simulink model "KUKA_AdaptiveComputedTorque"  (R2021a)
settings: Solver=FixedStepAuto  StartTime=0.0  StopTime=4  FixedStep=0.001  RelTol=1e-3
InitFcn:
  | Gamma=eye(8)*0.1;
  | K=[8100 900 6400 6400;180 60 160 160];
values from neighbouring files (symbols this model uses):
  m = {0 0 0 0 0}    [DynMatrixCalculator.m]
  N = {zeros(3,1) zeros(3,1) zeros(3,1) zeros(3,1) zeros(3,1)}    [DynMatrixCalculator.m]
undefined symbols (not defined in the file or in its folder): X, Y, Z
libraries: nesl_utility x17, sm_lib x16
(part 2 of 2)

== matlab function KUKA_AdaptiveComputedTorque/MATLAB Function1 ==
  data: Gamma input; K input; Theta_dd_ref input; Error input; Error_d input; Theta_dd input; Theta_d input; Theta input; Phi input; Tau output; Phi_hat_d output
function [Tau,Phi_hat_d] = Controller(Gamma,K,Theta_dd_ref, Error,Error_d,Theta_dd,Theta_d,Theta,Phi)

%% Input Data
d=Theta(1);
th2=Theta(2);
th3=Theta(3);
th4=Theta(4);

d_dt=Theta_d(1);
th2_dt=Theta_d(2);
th3_dt=Theta_d(3);
th4_dt=Theta_d(4);

d_ddt=Theta_dd(1);
th2_ddt=Theta_dd(2);
th3_ddt=Theta_dd(3);
th4_ddt=Theta_dd(4);


m1=Phi(1);m2=Phi(2);m3=Phi(3);m4=Phi(4);
I1=Phi(5);I2=Phi(6);I3=Phi(7);I4=Phi(8);
%% Params
g=9.80665;
% Kp = diag([100 100 100 100]);
% % ki = diag([2 4 4 4]);
% Kv = diag([20 20 20 20]);

Kp=diag(K(1,:));
% Ki=diag(K(2,:));
Kv=diag(K(2,:));

%% MVG
M =[                                                                                                                                                                                                                                                                                                                                                                                                        m1 + m2 + m3 + m4, (m2*cos(th2))/200 - (m2*sin(th2))/1000 + (m3*sin(th2))/1000 + (m4*sin(th2))/1000 + (11*m3*cos(th2)*cos(th3))/1000 + (59*m3*cos(th2)*sin(th3))/500 + (29*m4*cos(th2)*sin(th3))/100 - (143*m4*cos(th2)*cos(th3)*cos(th4))/1000 + (3*m4*cos(th2)*cos(th3)*sin(th4))/200 + (3*m4*cos(th2)*cos(th4)*sin(th3))/200 + (143*m4*cos(th2)*sin(th3)*sin(th4))/1000,                                                                                                                              sin(th2)*((59*m3*cos(th3))/500 + (29*m4*cos(th3))/100 - (11*m3*sin(th3))/1000 + (3*m4*cos(th3 + th4))/200 + (143*m4*sin(th3 + th4))/1000),             (20674^(1/2)*m4*sin(atan(15/143) + th3 + th4)*sin(th2))/1000
(m2*cos(th2))/200 - (m2*sin(th2))/1000 + (m3*sin(th2))/1000 + (m4*sin(th2))/1000 + (11*m3*cos(th2)*cos(th3))/1000 + (59*m3*cos(th2)*sin(th3))/500 + (29*m4*cos(th2)*sin(th3))/100 - (143*m4*cos(th2)*cos(th3)*cos(th4))/1000 + (3*m4*cos(th2)*cos(th3)*sin(th4))/200 + (3*m4*cos(th2)*cos(th4)*sin(th3))/200 + (143*m4*cos(th2)*sin(th3)*sin(th4))/1000,                 I2 + I3 + I4 + (13*m2)/500000 + (14047*m3)/2000000 + (13097*m4)/250000 + (87*m4*cos(th4))/20000 + (158*m4*cos(2*th3 + 2*th4))/15625 + (4147*m4*sin(th4))/100000 - (429*m4*sin(2*th3 + 2*th4))/200000 - (13803*m3*cos(2*th3))/2000000 - (841*m4*cos(2*th3))/20000 + (649*m3*sin(2*th3))/500000 - (87*m4*cos(2*th3 + th4))/20000 - (4147*m4*sin(2*th3 + th4))/100000, cos(th3)*((59*m3)/500000 + (m4*cos(th4)*((29*cos(th4))/100 + 3/200))/1000 + (m4*sin(th4)*((29*sin(th4))/100 + 143/1000))/1000) - sin(th3)*((11*m3)/1000000 + (m4*sin(th4)*((29*cos(th4))/100 + 3/200))/1000 - (m4*cos(th4)*((29*sin(th4))/100 + 143/1000))/1000),                      (20674^(1/2)*m4*sin(atan(15/143) + th3 + th4))/1000000
                                                                                                                                                                                                                                                                              (sin(th2)*(118*m3*cos(th3) + 290*m4*cos(th3) - 11*m3*sin(th3) + 15*m4*cos(th3 + th4) + 143*m4*sin(th3 + th4)))/1000,                                                                                                                                                                                                                                                        (59*m3*cos(th3))/500000 + (29*m4*cos(th3))/100000 - (11*m3*sin(th3))/1000000 + (3*m4*cos(th3 + th4))/200000 + (143*m4*sin(th3 + th4))/1000000,                                                                                                                                                                                       I3 + I4 + (2809*m3)/200000 + (52387*m4)/500000 + (87*m4*cos(th4))/10000 + (4147*m4*sin(th4))/50000, I4 + (10337*m4)/500000 + (87*m4*cos(th4))/20000 + (4147*m4*sin(th4))/100000
                                                                                                                                                                                                                                                                                                                                                    (20674^(1/2)*m4*sin(atan(15/143) + th3 + th4)*sin(th2))/1000,                                                                                                                                                                                                                                                                                                                                                (3*m4*cos(th3 + th4))/200000 + (143*m4*sin(th3 + th4))/1000000,                                                                                                                                                                                                              I4 + (10337*m4)/500000 + (87*m4*cos(th4))/20000 + (4147*m4*sin(th4))/100000,                                                            I4 + (10337*m4)/500000];

G =[                                                                                                                                                            0
                                                                                                                                                            0
(143*g*m4*cos(th3 + th4))/1000 - (59*g*m3*sin(th3))/500 - (29*g*m4*sin(th3))/100 - (11*g*m3*cos(th3))/1000 - (3*g*m4*sin(th3 + th4))/200
                                                                                                  (20674^(1/2)*g*m4*cos(atan(15/143) + th3 + th4))/1000];
 

                                                                                                  
W=[d_ddt, d_ddt + (th2_ddt*cos(th2))/200 - (th2_ddt*sin(th2))/1000 - (th2_dt^2*cos(th2))/1000 - (th2_dt^2*sin(th2))/200,                     d_ddt + (th2_ddt*sin(th2))/1000 + (th2_dt^2*cos(th2))/1000 + (11*th2_ddt*cos(th2)*cos(th3))/1000 + (59*th2_ddt*cos(th2)*sin(th3))/500 + (59*th3_ddt*cos(th3)*sin(th2))/500 - (11*th3_ddt*sin(th2)*sin(th3))/1000 - (11*th2_dt^2*cos(th3)*sin(th2))/1000 - (11*th3_dt^2*cos(th3)*sin(th2))/1000 - (59*th2_dt^2*sin(th2)*sin(th3))/500 - (59*th3_dt^2*sin(th2)*sin(th3))/500 + (59*th2_dt*th3_dt*cos(th2)*cos(th3))/250 - (11*th2_dt*th3_dt*cos(th2)*sin(th3))/500, d_ddt + (th2_ddt*sin(th2))/1000 + (th2_dt^2*cos(th2))/1000 + (29*th2_ddt*cos(th2)*sin(th3))/100 + (29*th3_ddt*cos(th3)*sin(th2))/100 - (29*th2_dt^2*sin(th2)*sin(th3))/100 - (29*th3_dt^2*sin(th2)*sin(th3))/100 - (3*th3_ddt*sin(th2)*sin(th3)*sin(th4))/200 - (3*th4_ddt*sin(th2)*sin(th3)*sin(th4))/200 + (143*th2_dt^2*cos(th3)*cos(th4)*sin(th2))/1000 + (143*th3_dt^2*cos(th3)*cos(th4)*sin(th2))/1000 + (143*th4_dt^2*cos(th3)*cos(th4)*sin(th2))/1000 - (3*th2_dt^2*cos(th3)*sin(th2)*sin(th4))/200 - (3*th2_dt^2*cos(th4)*sin(th2)*sin(th3))/200 - (3*th3_dt^2*cos(th3)*sin(th2)*sin(th4))/200 - (3*th3_dt^2*cos(th4)*sin(th2)*sin(th3))/200 - (3*th4_dt^2*cos(th3)*sin(th2)*sin(th4))/200 - (3*th4_dt^2*cos(th4)*sin(th2)*sin(th3))/200 - (143*th2_dt^2*sin(th2)*sin(th3)*sin(th4))/1000 - (143*th3_dt^2*sin(th2)*sin(th3)*sin(th4))/1000 - (143*th4_dt^2*sin(th2)*sin(th3)*sin(th4))/1000 + (29*th2_dt*th3_dt*cos(th2)*cos(th3))/50 - (143*th2_ddt*cos(th2)*cos(th3)*cos(th4))/1000 + (3*th2_ddt*cos(th2)*cos(th3)*sin(th4))/200 + (3*th2_ddt*cos(th2)*cos(th4)*sin(th3))/200 + (3*th3_ddt*cos(th3)*cos(th4)*sin(th2))/200 + (3*th4_ddt*cos(th3)*cos(th4)*sin(th2))/200 + (143*th2_ddt*cos(th2)*sin(th3)*sin(th4))/1000 + (143*th3_ddt*cos(th3)*sin(th2)*sin(th4))/1000 + (143*th3_ddt*cos(th4)*sin(th2)*sin(th3))/1000 + (143*th4_ddt*cos(th3)*sin(th2)*sin(th4))/1000 + (143*th4_ddt*cos(th4)*sin(th2)*sin(th3))/1000 + (3*th2_dt*th3_dt*cos(th2)*cos(th3)*cos(th4))/100 + (3*th2_dt*th4_dt*cos(th2)*cos(th3)*cos(th4))/100 + (143*th2_dt*th3_dt*cos(th2)*cos(th3)*sin(th4))/500 + (143*th2_dt*th3_dt*cos(th2)*cos(th4)*sin(th3))/500 + (143*th2_dt*th4_dt*cos(th2)*cos(th3)*sin(th4))/500 + (143*th2_dt*th4_dt*cos(th2)*cos(th4)*sin(th3))/500 + (143*th3_dt*th4_dt*cos(th3)*cos(th4)*sin(th2))/500 - (3*th2_dt*th3_dt*cos(th2)*sin(th3)*sin(th4))/100 - (3*th2_dt*th4_dt*cos(th2)*sin(th3)*sin(th4))/100 - (3*th3_dt*th4_dt*cos(th3)*sin(th2)*sin(th4))/100 - (3*th3_dt*th4_dt*cos(th4)*sin(th2)*sin(th3))/100 - (143*th3_dt*th4_dt*sin(th2)*sin(th3)*sin(th4))/500, 0,      0,      0,               0
     0,                                        (13*th2_ddt)/500000 + (d_ddt*cos(th2))/200 - (d_ddt*sin(th2))/1000, (14047*th2_ddt)/2000000 + (11*d_ddt*cos(th2 + th3))/2000 + (59*d_ddt*sin(th2 + th3))/1000 + (59*th3_ddt*cos(th3))/500000 + (d_ddt*sin(th2))/1000 - (11*th3_ddt*sin(th3))/1000000 + (11*d_ddt*cos(th2 - th3))/2000 - (59*d_ddt*sin(th2 - th3))/1000 - (13803*th2_ddt*cos(2*th3))/2000000 - (11*th3_dt^2*cos(th3))/1000000 + (649*th2_ddt*sin(2*th3))/500000 - (59*th3_dt^2*sin(th3))/500000 + (649*th2_dt*th3_dt*cos(2*th3))/250000 + (13803*th2_dt*th3_dt*sin(2*th3))/1000000,                                                                                                                                                                                                                                                                                                                                                                                                                                                                                                                                             (13097*th2_ddt)/250000 + (3*th3_ddt*cos(th3 + th4))/200000 + (3*th4_ddt*cos(th3 + th4))/200000 + (29*d_ddt*sin(th2 + th3))/200 + (143*th3_ddt*sin(th3 + th4))/1000000 + (143*th4_ddt*sin(th3 + th4))/1000000 + (87*th2_ddt*cos(th4))/20000 + (29*th3_ddt*cos(th3))/100000 - (143*d_ddt*cos(th2 + th3 + th4))/2000 + (d_ddt*sin(th2))/1000 + (4147*th2_ddt*sin(th4))/100000 - (87*th2_ddt*cos(2*th3 + th4))/20000 + (143*th3_dt^2*cos(th3 + th4))/1000000 + (143*th4_dt^2*cos(th3 + th4))/1000000 + (3*d_ddt*sin(th2 + th3 + th4))/400 - (29*d_ddt*sin(th2 - th3))/200 - (4147*th2_ddt*sin(2*th3 + th4))/100000 - (3*th3_dt^2*sin(th3 + th4))/200000 - (3*th4_dt^2*sin(th3 + th4))/200000 - (841*th2_ddt*cos(2*th3))/20000 - (143*d_ddt*cos(th3 - th2 + th4))/2000 - (29*th3_dt^2*sin(th3))/100000 + (158*th2_ddt*cos(2*th3 + 2*th4))/15625 + (3*d_ddt*sin(th3 - th2 + th4))/400 - (429*th2_ddt*sin(2*th3 + 2*th4))/200000 + (841*th2_dt*th3_dt*sin(2*th3))/10000 - (429*th2_dt*th3_dt*cos(2*th3 + 2*th4))/100000 - (429*th2_dt*th4_dt*cos(2*th3 + 2*th4))/100000 - (316*th2_dt*th3_dt*sin(2*th3 + 2*th4))/15625 - (316*th2_dt*th4_dt*sin(2*th3 + 2*th4))/15625 + (143*th3_dt*th4_dt*cos(th3 + th4))/500000 - (3*th3_dt*th4_dt*sin(th3 + th4))/100000 + (4147*th2_dt*th4_dt*cos(th4))/100000 - (87*th2_dt*th4_dt*sin(th4))/20000 - (4147*th2_dt*th3_dt*cos(2*th3 + th4))/50000 - (4147*th2_dt*th4_dt*cos(2*th3 + th4))/100000 + (87*th2_dt*th3_dt*sin(2*th3 + th4))/10000 + (87*th2_dt*th4_dt*sin(2*th3 + th4))/20000, 0, th2_ddt, th2_ddt,          th2_ddt
     0,                                                                                                          0,                                                                                                                                                                                          (2809*th3_ddt)/200000 - (649*th2_dt^2*cos(2*th3))/500000 - (13803*th2_dt^2*sin(2*th3))/2000000 + (59*th2_ddt*cos(th3))/500000 - (11*th2_ddt*sin(th3))/1000000 - (11*g*cos(th3))/1000 - (59*g*sin(th3))/500 + (59*d_ddt*cos(th3)*sin(th2))/500 - (11*d_ddt*sin(th2)*sin(th3))/1000,                                                                                                                                                                                                                                                                                                                                                                                                                                                                                                                                                                                                                                                                                                                                                                                                                                                                                                                                                                                                                                                                                                                                                                                               (52387*th3_ddt)/500000 + (10337*th4_ddt)/500000 + (3*th2_ddt*cos(th3 + th4))/200000 + (143*th2_ddt*sin(th3 + th4))/1000000 + (143*g*cos(th3 + th4))/1000 - (841*th2_dt^2*sin(2*th3))/20000 + (429*th2_dt^2*cos(2*th3 + 2*th4))/200000 - (3*g*sin(th3 + th4))/200 + (158*th2_dt^2*sin(2*th3 + 2*th4))/15625 + (29*th2_ddt*cos(th3))/100000 + (87*th3_ddt*cos(th4))/10000 + (87*th4_ddt*cos(th4))/20000 + (4147*th3_ddt*sin(th4))/50000 + (4147*th4_ddt*sin(th4))/100000 - (29*g*sin(th3))/100 + (4147*th4_dt^2*cos(th4))/100000 - (87*th4_dt^2*sin(th4))/20000 + (4147*th2_dt^2*cos(2*th3 + th4))/100000 - (87*th2_dt^2*sin(2*th3 + th4))/20000 + (29*d_ddt*cos(th3)*sin(th2))/100 + (4147*th3_dt*th4_dt*cos(th4))/50000 - (87*th3_dt*th4_dt*sin(th4))/10000 + (3*d_ddt*cos(th3 + th4)*sin(th2))/200 + (143*d_ddt*sin(th3 + th4)*sin(th2))/1000, 0,      0, th3_ddt, th3_ddt + th4_ddt
     0,                                                                                                          0,                                                                                                                                                                                                                                                                                                                                                                                                                                                                       0,                                                                                                                                                                                                                                                                                                                                                                                                                                                                                                                                                                                                                                                                                                                                                                                                                                                                                                                                                                                                                                                                                                                                                                                                                                                                                                                                                                                                                                            (10337*th4_ddt)/500000 + (429*th2_dt^2*cos(2*th3 + 2*th4))/200000 + (158*th2_dt^2*sin(2*th3 + 2*th4))/15625 + th3_ddt*((87*cos(th4))/20000 + (4147*sin(th4))/100000 + 10337/500000) + (th2_ddt*(15*cos(th3 + th4) + 143*sin(th3 + th4)))/1000000 - (4147*th2_dt^2*cos(th4))/200000 - (4147*th3_dt^2*cos(th4))/100000 + (87*th2_dt^2*sin(th4))/40000 + (87*th3_dt^2*sin(th4))/20000 + (4147*th2_dt^2*cos(2*th3 + th4))/200000 - (87*th2_dt^2*sin(2*th3 + th4))/40000 + (20674^(1/2)*g*cos(th3 + th4 + atan(15/143)))/1000 + (20674^(1/2)*d_ddt*sin(th2)*sin(th3 + th4 + atan(15/143)))/1000, 0,      0,      0, th3_ddt + th4_ddt];


Vm=[-(th2_dt^2*m2*cos(th2) - th2_dt^2*m3*cos(th2) - th2_dt^2*m4*cos(th2) + 5*th2_dt^2*m2*sin(th2) + 118*th2_dt^2*m3*sin(th2)*sin(th3) + 290*th2_dt^2*m4*sin(th2)*sin(th3) + 118*th3_dt^2*m3*sin(th2)*sin(th3) + 290*th3_dt^2*m4*sin(th2)*sin(th3) + 11*th2_dt^2*m3*cos(th3)*sin(th2) + 11*th3_dt^2*m3*cos(th3)*sin(th2) - 143*th2_dt^2*m4*cos(th3)*cos(th4)*sin(th2) - 143*th3_dt^2*m4*cos(th3)*cos(th4)*sin(th2) - 143*th4_dt^2*m4*cos(th3)*cos(th4)*sin(th2) + 15*th2_dt^2*m4*cos(th3)*sin(th2)*sin(th4) + 15*th2_dt^2*m4*cos(th4)*sin(th2)*sin(th3) + 15*th3_dt^2*m4*cos(th3)*sin(th2)*sin(th4) + 15*th3_dt^2*m4*cos(th4)*sin(th2)*sin(th3) + 15*th4_dt^2*m4*cos(th3)*sin(th2)*sin(th4) + 15*th4_dt^2*m4*cos(th4)*sin(th2)*sin(th3) + 143*th2_dt^2*m4*sin(th2)*sin(th3)*sin(th4) + 143*th3_dt^2*m4*sin(th2)*sin(th3)*sin(th4) + 143*th4_dt^2*m4*sin(th2)*sin(th3)*sin(th4) - 236*th2_dt*th3_dt*m3*cos(th2)*cos(th3) - 580*th2_dt*th3_dt*m4*cos(th2)*cos(th3) + 22*th2_dt*th3_dt*m3*cos(th2)*sin(th3) - 30*th2_dt*th3_dt*m4*cos(th2)*cos(th3)*cos(th4) - 30*th2_dt*th4_dt*m4*cos(th2)*cos(th3)*cos(th4) - 286*th2_dt*th3_dt*m4*cos(th2)*cos(th3)*sin(th4) - 286*th2_dt*th3_dt*m4*cos(th2)*cos(th4)*sin(th3) - 286*th2_dt*th4_dt*m4*cos(th2)*cos(th3)*sin(th4) - 286*th2_dt*th4_dt*m4*cos(th2)*cos(th4)*sin(th3) - 286*th3_dt*th4_dt*m4*cos(th3)*cos(th4)*sin(th2) + 30*th2_dt*th3_dt*m4*cos(th2)*sin(th3)*sin(th4) + 30*th2_dt*th4_dt*m4*cos(th2)*sin(th3)*sin(th4) + 30*th3_dt*th4_dt*m4*cos(th3)*sin(th2)*sin(th4) + 30*th3_dt*th4_dt*m4*cos(th4)*sin(th2)*sin(th3) + 286*th3_dt*th4_dt*m4*sin(th2)*sin(th3)*sin(th4))/(1000*(d_dt+0.0001)), 0, 0, 0
                                                                                                                                                                                                                                                                                                                                                                                                                                                                                                                                                                                                                                                                                                                                                                     -(11*th3_dt^2*m3*cos(th3) + 118*th3_dt^2*m3*sin(th3) + 290*th3_dt^2*m4*sin(th3) - 143*th3_dt^2*m4*cos(th3 + th4) - 143*th4_dt^2*m4*cos(th3 + th4) + 15*th3_dt^2*m4*sin(th3 + th4) + 15*th4_dt^2*m4*sin(th3 + th4) - 41470*th2_dt*th4_dt*m4*cos(th4) + 4350*th2_dt*th4_dt*m4*sin(th4) + 82940*th2_dt*th3_dt*m4*cos(2*th3 + th4) + 41470*th2_dt*th4_dt*m4*cos(2*th3 + th4) - 8700*th2_dt*th3_dt*m4*sin(2*th3 + th4) - 4350*th2_dt*th4_dt*m4*sin(2*th3 + th4) - 2596*th2_dt*th3_dt*m3*cos(2*th3) - 13803*th2_dt*th3_dt*m3*sin(2*th3) - 84100*th2_dt*th3_dt*m4*sin(2*th3) + 4290*th2_dt*th3_dt*m4*cos(2*th3 + 2*th4) + 4290*th2_dt*th4_dt*m4*cos(2*th3 + 2*th4) + 20224*th2_dt*th3_dt*m4*sin(2*th3 + 2*th4) + 20224*th2_dt*th4_dt*m4*sin(2*th3 + 2*th4) - 286*th3_dt*th4_dt*m4*cos(th3 + th4) + 30*th3_dt*th4_dt*m4*sin(th3 + th4))/(1000000*(d_dt+0.0001)), 0, 0, 0
                                                                                                                                                                                                                                                                                                                                                                                                                                                                                                                                                                                                                                                                                                                                                                                                                                                                                                                                                                                                                                                                                                                                                                                            -(8700*th4_dt^2*m4*sin(th4) - 82940*th4_dt^2*m4*cos(th4) - 82940*th2_dt^2*m4*cos(2*th3 + th4) + 8700*th2_dt^2*m4*sin(2*th3 + th4) + 2596*th2_dt^2*m3*cos(2*th3) + 13803*th2_dt^2*m3*sin(2*th3) + 84100*th2_dt^2*m4*sin(2*th3) - 4290*th2_dt^2*m4*cos(2*th3 + 2*th4) - 20224*th2_dt^2*m4*sin(2*th3 + 2*th4) - 165880*th3_dt*th4_dt*m4*cos(th4) + 17400*th3_dt*th4_dt*m4*sin(th4))/(2000000*(d_dt+0.0001)), 0, 0, 0
                                                                                                                                                                                                                                                                                                                                                                                                                                                                                                                                                                                                                                                                                                                                                                                                                                                                                                                                                                                                                                                                                                                                                                                                                                                                                                (2175*th2_dt^2*m4*sin(th4) - 41470*th3_dt^2*m4*cos(th4) - 20735*th2_dt^2*m4*cos(th4) + 4350*th3_dt^2*m4*sin(th4) + 20735*th2_dt^2*m4*cos(2*th3 + th4) - 2175*th2_dt^2*m4*sin(2*th3 + th4) + 2145*th2_dt^2*m4*cos(2*th3 + 2*th4) + 10112*th2_dt^2*m4*sin(2*th3 + 2*th4))/(1000000*(d_dt+0.0001)), 0, 0, 0];
 
E=[Error;Error_d];
B=[zeros(4,4);ones(4,4)];
% A=[zeros(4,4) ones(4,4);-Kp -Kv];
P=[(Kp+Kv/2)*ones(4,4) ones(4,4)/2;ones(4,4)/2 ones(4,4)]/2;
% Q=-(A'*P+P*A);
Phi_hat_d=Gamma*W'*(M^-1)*B'*P*E;
Tau=M*(Theta_dd_ref+Kv*Error_d+Kp*Error)+Vm*Theta_d+G;

end

== matlab function KUKA_AdaptiveComputedTorque/Trajectory/MATLAB Function ==
  data: time input; d output; th2 output; th3 output; th4 output; d_dt output; th2_dt output; th3_dt output; th4_dt output; d_ddt output; th2_ddt output; th3_ddt output; th4_ddt output
function [d,th2,th3,th4,d_dt,th2_dt,th3_dt,th4_dt,d_ddt,th2_ddt,th3_ddt,th4_ddt] = fcn(time)
time=time*5;
d=  (1/4)*(1-cos(time*pi/5));
th2= (pi/4)*(1-cos(time*pi/5));
th3= -(pi/4)*(1-cos(time*pi/5));
th4=  (pi/4)*(1-cos(time*pi/5));

d_dt= (pi/20)*sin(time*pi/5);
th2_dt=(pi^2/20)*sin(time*pi/5);
th3_dt=-(pi^2/20)*sin(time*pi/5);
th4_dt= (pi^2/20)*sin(time*pi/5);

d_ddt= (pi^2/100)*cos(time*pi/5);
th2_ddt=(pi^3/100)*cos(time*pi/5);
th3_ddt=-(pi^3/100)*cos(time*pi/5);
th4_ddt= (pi^3/100)*cos(time*pi/5);
